simulink model "mapTest"  (R2019b)
settings: Solver=FixedStepAuto  StartTime=0.0  StopTime=1  FixedStep=.001  RelTol=1e-3
libraries: Map x1
settings Model: Creator=Nick  LastModifiedBy=Nick

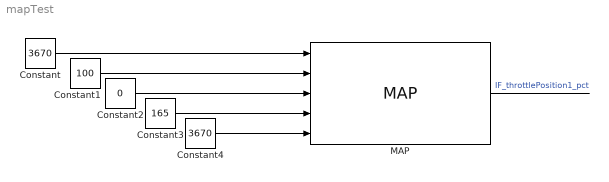
== system mapTest ==
  Constant : Constant  Value=3670
  Constant1 : Constant  Value=100
  Constant2 : Constant  Value=0
  Constant3 : Constant  Value=165
  Constant4 : Constant  Value=3670
  MAP : Map/Algroithms/MAP  SystemSampleTime=-1  Latency=0  AutoFrameSizeCalculation=off
  wires:
  MAP/1 -> ?  "IF_throttlePosition1_pct"
  Constant/1 -> MAP/1
  Constant1/1 -> MAP/2
  Constant2/1 -> MAP/3
  Constant4/1 -> MAP/5
  Constant3/1 -> MAP/4
